simulink library "CRYP_TM_MASTER"  (Simulink 8.6)
settings: Solver=ode45  StartTime=0.0  StopTime=10.0  RelTol=1e-3
libraries: cdsEpicsOut x49, cdsTP x16, VIS_LIB x11, cdsFilt x5, cdsFunctionCall x5, cdsEpicsBinIn x4, cdsFiltCtrl x4, CRYP_TM_MASTER x4, cdsMuxMatrix x3, QPD x2, KAGRA_UTIL x1, cdsEpicsIn x1
(part 1 of 2)
settings Model: Creator=controls  LastModifiedBy=controls

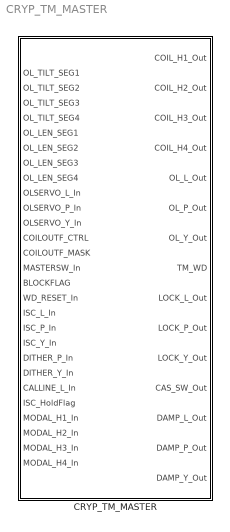
== system CRYP_TM_MASTER ==
  CRYP_TM_MASTER : Subsystem

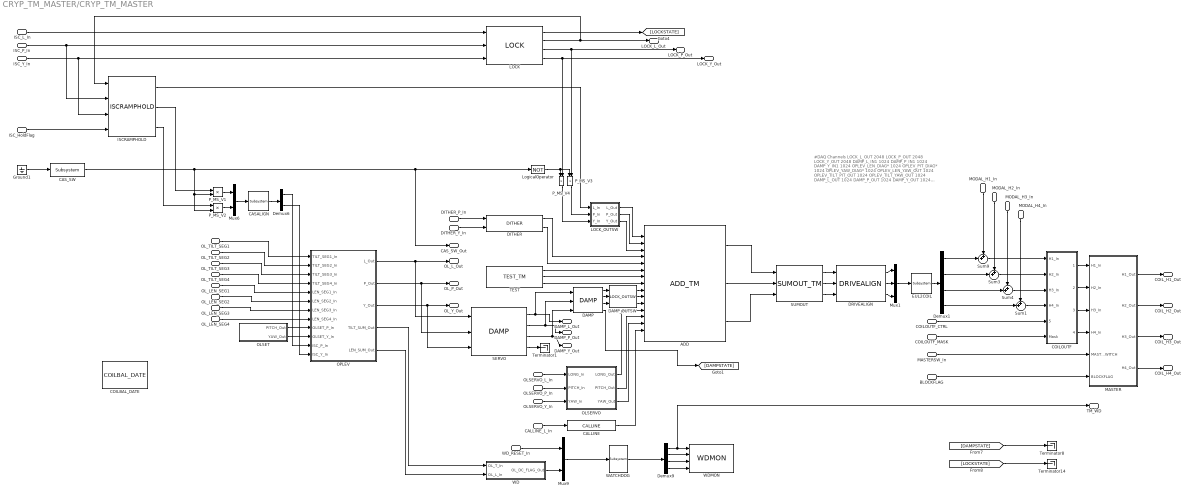
== system CRYP_TM_MASTER/CRYP_TM_MASTER ==
  note: #DAQ Channels
      | LOCK_L_OUT 2048
      | LOCK_P_OUT 2048
      | LOCK_Y_OUT 2048
      | DAMP_L_IN1 1024
      | DAMP_P_IN1 1024
      | DAMP_Y_IN1 1024
      | OPLEV_LEN_DIAG* 1024
      | OPLEV_PIT_DIAG* 1024
      | OPLEV_YAW_DIAG* 1024
      | OPLEV_LEN_YAW_OUT 1024
      | OPLEV_TILT_PIT_OUT 1024
      | OPLEV_TILT_YAW_OUT 1024
      | DAMP_L_OUT 1024
      | DAMP_P_OUT 1024
      | DAMP_Y_OUT 1024
      | MASTER_OUT_H1 1024
      | MASTER_OUT_H2 1024
      | MASTER_OUT_H3 1024
      | MASTER_OUT_H4 1024
      | SUMOUT_L_OUT 512
      | SUMOUT_P_OUT 512
      | SUMOUT_Y_OUT 512
  OL_TILT_SEG1 : Inport
  OL_TILT_SEG2 : Inport  Port=2
  OL_TILT_SEG3 : Inport  Port=3
  OL_TILT_SEG4 : Inport  Port=4
  OL_LEN_SEG1 : Inport  Port=5
  OL_LEN_SEG2 : Inport  Port=6
  OL_LEN_SEG3 : Inport  Port=7
  OL_LEN_SEG4 : Inport  Port=8
  OLSERVO_L_In : Inport  Port=9
  OLSERVO_P_In : Inport  Port=10
  OLSERVO_Y_In : Inport  Port=11
  COILOUTF_CTRL : Inport  Port=12
  COILOUTF_MASK : Inport  Port=13
  MASTERSW_In : Inport  Port=14
  BLOCKFLAG : Inport  Port=15
  WD_RESET_In : Inport  Port=16
  ISC_L_In : Inport  Port=17
  ISC_P_In : Inport  Port=18
  ISC_Y_In : Inport  Port=19
  DITHER_P_In : Inport  Port=20
  DITHER_Y_In : Inport  Port=21
  CALLINE_L_In : Inport  Port=22
  ISC_HoldFlag : Inport  Port=23
  MODAL_H1_In : Inport  Port=24
  MODAL_H2_In : Inport  Port=25
  MODAL_H3_In : Inport  Port=26
  MODAL_H4_In : Inport  Port=27
  ADD : VIS_LIB/CrypParts/ADD_TM
  CALLINE : VIS_LIB/CALLINE
  CASALIGN : cdsMuxMatrix/Subsystem  Tag=cdsMuxMatrix  Description=Any size matrix. Inputs and outputs must be connected using Mux and Demux parts.
      settings: AttributesFormatString=%<Tag>
  CAS_SW : cdsEpicsBinIn/Subsystem  Tag=cdsEpicsBinIn  Description=|
      | Purpose:                                                                            
      | Create an EPICS binary (0 or 1) input channel to the FE realtime controls.          
      |                                                                                     
      | Operation:                                                                          
      | Outputs value from an EPICS ai record. Value is binary input (bi Epics record type).
      |                                                                                     
      | Usage:                                                                              
      | Name the part with the desired EPICS channel name.
      settings: AttributesFormatString=%<Tag>
  COILBAL_DATE : VIS_LIB/COILBAL_DATE
  COILOUTF : Subsystem
  DAMP : VIS_LIB/DAMP
  DAMP_OUTSW : CRYP_TM_MASTER/CRYP_TM_MASTER/LOCK_OUTSW
  DITHER : VIS_LIB/DITHER
  DRIVEALIGN : VIS_LIB/CrypParts/DRIVEALIGN
  Demux1 : Demux
  Demux6 : Demux  Outputs=2
  Demux9 : Demux
  EUL2COIL : cdsMuxMatrix/Subsystem  Tag=cdsMuxMatrix  Description=Any size matrix. Inputs and outputs must be connected using Mux and Demux parts.
      settings: AttributesFormatString=%<Tag>
  Ground1 : Ground
  ISCRAMPHOLD : KAGRA_UTIL/ISCRAMPHOLD
  LOCK : VIS_LIB/LOCK
  LOCK_OUTSW : Subsystem
  LogicalOperator : Logic  Operator=NOT  AllPortsSameDT=off  OutDataTypeStr=boolean
  MASTER : Subsystem
  Mux1 : Mux  Inputs=3
  Mux6 : Mux  Inputs=2
  Mux9 : Mux  Inputs=2
  OLSERVO : Subsystem
  OLSET : Subsystem
  OPLEV : Subsystem
  P_MS_V{1..4} (4 alike) : Product  RndMeth=Zero
  SERVO : VIS_LIB/DAMP
  SUMOUT : VIS_LIB/CrypParts/SUMOUT_TM
  Sum{1,3..4,9} (4 alike) : Sum  Inputs=++|
  TEST : VIS_LIB/CrypParts/TEST_TM
  Terminator1 : Terminator
  Terminator14 : Terminator
  Terminator8 : Terminator
  WATCHDOG : cdsFunctionCall/Subsystem  Tag=cdsFunctionCall  Description=inline OSEMWATCHDOG /opt/rtcds/userapps/release/vis/common/src/WATCHDOG.c
      settings: AttributesFormatString=%<Tag>\n%<Description>
  WD : Subsystem
  WDMON : VIS_LIB/WDMON
  COIL_H1_Out : Outport
  COIL_H2_Out : Outport  Port=2
  COIL_H3_Out : Outport  Port=3
  COIL_H4_Out : Outport  Port=4
  OL_L_Out : Outport  Port=5
  OL_P_Out : Outport  Port=6
  OL_Y_Out : Outport  Port=7
  TM_WD : Outport  Port=8
  LOCK_L_Out : Outport  Port=9
  LOCK_P_Out : Outport  Port=10
  LOCK_Y_Out : Outport  Port=11
  CAS_SW_Out : Outport  Port=12
  DAMP_L_Out : Outport  Port=13
  DAMP_P_Out : Outport  Port=14
  DAMP_Y_Out : Outport  Port=15
  wires:
  ADD/3 -> SUMOUT/3
  ADD/2 -> SUMOUT/2
  ADD/1 -> SUMOUT/1
  Demux1/4 -> Sum1/2
  MODAL_H4_In/1 -> Sum1/1
  Sum1/1 -> COILOUTF/4(H4_In)
  Demux1/3 -> Sum4/2
  Demux1/2 -> Sum3/2
  MODAL_H3_In/1 -> Sum4/1
  Sum4/1 -> COILOUTF/3(H3_In)
  MODAL_H2_In/1 -> Sum3/1
  Sum3/1 -> COILOUTF/2(H2_In)
  Demux1/1 -> Sum9/2
  MODAL_H1_In/1 -> Sum9/1
  Sum9/1 -> COILOUTF/1(H1_In)
  ISC_P_In/1 -> LOCK/2, ISCRAMPHOLD/2
  ISCRAMPHOLD/1 -> LOCK_OUTSW/1(L_In)
  ISCRAMPHOLD/3 -> P_MS_V2/1
  ISCRAMPHOLD/2 -> P_MS_V1/1
  ISC_HoldFlag/1 -> ISCRAMPHOLD/4
  ISC_Y_In/1 -> LOCK/3, ISCRAMPHOLD/3
  LOCK/2 -> ISCRAMPHOLD/1, LOCK_L_Out/1
  OL_TILT_SEG3/1 -> OPLEV/3(TILT_SEG3_In)
  OL_LEN_SEG4/1 -> OPLEV/8(LEN_SEG4_In)
  OL_LEN_SEG3/1 -> OPLEV/7(LEN_SEG3_In)
  OL_LEN_SEG2/1 -> OPLEV/6(LEN_SEG2_In)
  OL_LEN_SEG1/1 -> OPLEV/5(LEN_SEG1_In)
  OL_TILT_SEG4/1 -> OPLEV/4(TILT_SEG4_In)
  OL_TILT_SEG2/1 -> OPLEV/2(TILT_SEG2_In)
  OL_TILT_SEG1/1 -> OPLEV/1(TILT_SEG1_In)
  COILOUTF_CTRL/1 -> COILOUTF/5(Control)
  COILOUTF_MASK/1 -> COILOUTF/6(Mask)
  WD_RESET_In/1 -> Mux9/1
  COILOUTF/4(H4_Out) -> MASTER/4(H4_In)
  COILOUTF/3(H3_Out) -> MASTER/3(H3_In)
  COILOUTF/2(H2_Out) -> MASTER/2(H2_In)
  COILOUTF/1(H1_Out) -> MASTER/1(H1_In)
  Demux9/1 -> TM_WD/1, WDMON/1
  Mux9/1 -> WATCHDOG/1
  WATCHDOG/1 -> Demux9/1
  Demux9/4 -> WDMON/4
  Demux9/3 -> WDMON/3
  Demux9/2 -> WDMON/2
  EUL2COIL/1 -> Demux1/1
  Mux1/1 -> EUL2COIL/1
  DITHER_P_In/1 -> DITHER/1
  DITHER_Y_In/1 -> DITHER/2
  MASTER/1(H1_Out) -> COIL_H1_Out/1
  MASTER/2(H2_Out) -> COIL_H2_Out/1
  MASTER/3(H3_Out) -> COIL_H3_Out/1
  MASTER/4(H4_Out) -> COIL_H4_Out/1
  MASTERSW_In/1 -> MASTER/5(MASTERSWITCH)
  [DAMPSTATE] -> Terminator8/1
  [LOCKSTATE] -> Terminator14/1
  LOCK/1 -> [LOCKSTATE]
  WD/1(OL_DC_FLAG_Out) -> Mux9/2
  ISC_L_In/1 -> LOCK/1
  BLOCKFLAG/1 -> MASTER/6(BLOCKFLAG)
  OPLEV/1(L_Out) -> SERVO/1, OL_L_Out/1
  OPLEV/2(P_Out) -> SERVO/2, OL_P_Out/1
  OPLEV/3(Y_Out) -> SERVO/3, OL_Y_Out/1
  OPLEV/4(TILT_SUM_Out) -> WD/1(OL_T_In)
  OPLEV/5(LEN_SUM_Out) -> WD/2(OL_L_In)
  LOCK/4 -> LOCK_Y_Out/1, P_MS_V4/2
  LOCK/3 -> LOCK_P_Out/1, P_MS_V3/2
  DITHER/2 -> ADD/5
  DITHER/1 -> ADD/4
  TEST/3 -> ADD/8
  TEST/2 -> ADD/7
  TEST/1 -> ADD/6
  SERVO/2 -> DAMP/2, DAMP_P_Out/1
  SERVO/3 -> DAMP/3, DAMP_Y_Out/1
  SUMOUT/2 -> DRIVEALIGN/2
  SUMOUT/1 -> DRIVEALIGN/1
  SUMOUT/3 -> DRIVEALIGN/3
  DRIVEALIGN/3 -> Mux1/3
  DRIVEALIGN/1 -> Mux1/1
  DRIVEALIGN/2 -> Mux1/2
  OLSERVO_L_In/1 -> OLSERVO/1(LONG_In)
  OLSERVO_P_In/1 -> OLSERVO/2(PITCH_In)
  OLSERVO_Y_In/1 -> OLSERVO/3(YAW_In)
  OLSERVO/1(LONG_Out) -> ADD/12
  OLSERVO/2(PITCH_Out) -> ADD/13
  OLSERVO/3(YAW_Out) -> ADD/14
  LOCK_OUTSW/1(L_Out) -> ADD/1
  LOCK_OUTSW/2(P_Out) -> ADD/2
  LOCK_OUTSW/3(Y_Out) -> ADD/3
  OLSET/1(PITCH_Out) -> OPLEV/9(OLSET_P_In)
  OLSET/2(YAW_Out) -> OPLEV/10(OLSET_Y_In)
  Ground1/1 -> CAS_SW/1
  P_MS_V1/1 -> Mux6/1
  P_MS_V2/1 -> Mux6/2
  Mux6/1 -> CASALIGN/1
  CASALIGN/1 -> Demux6/1
  Demux6/1 -> OPLEV/11(ISC_P_In)
  Demux6/2 -> OPLEV/12(ISC_Y_In)
  P_MS_V4/1 -> LOCK_OUTSW/3(Y_In)
  P_MS_V3/1 -> LOCK_OUTSW/2(P_In)
  LogicalOperator/1 -> P_MS_V4/1, P_MS_V3/1
  CAS_SW/1 -> P_MS_V2/2, P_MS_V1/2, CAS_SW_Out/1, LogicalOperator/1
  SERVO/1 -> DAMP/1, DAMP_L_Out/1
  DAMP_OUTSW/1 -> ADD/9
  DAMP_OUTSW/2 -> ADD/10
  DAMP_OUTSW/3 -> ADD/11
  SERVO/4 -> Terminator1/1
  DAMP/4 -> [DAMPSTATE]
  DAMP/1 -> DAMP_OUTSW/1
  DAMP/2 -> DAMP_OUTSW/2
  DAMP/3 -> DAMP_OUTSW/3
  CALLINE_L_In/1 -> CALLINE/1
  CALLINE/1 -> ADD/15

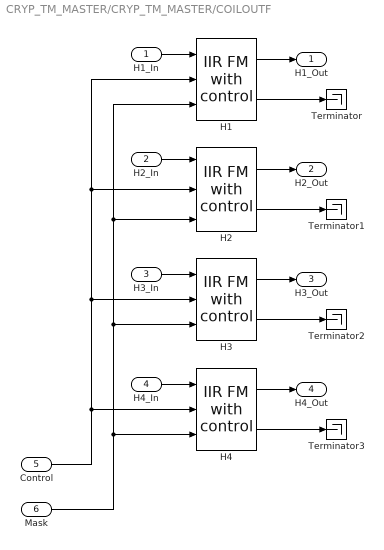
== system CRYP_TM_MASTER/CRYP_TM_MASTER/COILOUTF ==
  H1_In : Inport
  H2_In : Inport  Port=2
  H3_In : Inport  Port=3
  H4_In : Inport  Port=4
  Control : Inport  Port=5
  Mask : Inport  Port=6
  H1 : cdsFiltCtrl/IIR FM with control  Tag=cdsFiltCtrl  Description=|
      | cdsFiltCntrl is the standard IIR filter module (exactly the same as cdsFilt) but with added control data output 'Ctrl'. Filter module digital signal output appears on the first output, which is called 'Val'. 'Ctrl' output has a bit pattern encoding the state of filter's on/off switches (FM1 through FM10). The bit values are:
      |                                                                                                                                                                                                                                                                                                                                       
      | module 	hex	dec                                                                                                                                                                                                                                                                                                                       
      | -----------------------                                                                                                                                                                                                                                                                                                               
      | FM1	0x20                    32                                                                                                                                                                                                                                                                                                        
      | FM2	0x80                     128                                                                                                                                                                                                                                                                                                      
      | FM3	0x200                   512                                                                                                                                                                                                                                                                                                       
      | FM4	0x800                   2048                                                                                                                                                                                                                                                                                                      
      | FM5	0x2000                 8192                                                                                                                                                                                                                                                                                                       
      | FM6	0x8000                 32768                                                                                                                                                                                                                                                                                                      
      | FM7	0x20000                131072                                                                                                                                                                                                                                                                                                     
      | FM8	0x80000                 524288                                                                                                                                                                                                                                                                                                    
      | FM9	0x200000               2097152                                                                                                                                                                                                                                                                                                    
      | FM10	0x800000               8388608                                                                                                                                                                                                                                                                                                   
      |                                                                                                                                                                                                                                                                                                                                       
      | This bit data can be used to drive some other switches or it can be output using a binary I/O module.
      settings: AttributesFormatString=%<Tag>
  H2 : cdsFiltCtrl/IIR FM with control  Tag=cdsFiltCtrl  Description=|
      | cdsFiltCntrl is the standard IIR filter module (exactly the same as cdsFilt) but with added control data output 'Ctrl'. Filter module digital signal output appears on the first output, which is called 'Val'. 'Ctrl' output has a bit pattern encoding the state of filter's on/off switches (FM1 through FM10). The bit values are:
      |                                                                                                                                                                                                                                                                                                                                       
      | module 	hex	dec                                                                                                                                                                                                                                                                                                                       
      | -----------------------                                                                                                                                                                                                                                                                                                               
      | FM1	0x20                    32                                                                                                                                                                                                                                                                                                        
      | FM2	0x80                     128                                                                                                                                                                                                                                                                                                      
      | FM3	0x200                   512                                                                                                                                                                                                                                                                                                       
      | FM4	0x800                   2048                                                                                                                                                                                                                                                                                                      
      | FM5	0x2000                 8192                                                                                                                                                                                                                                                                                                       
      | FM6	0x8000                 32768                                                                                                                                                                                                                                                                                                      
      | FM7	0x20000                131072                                                                                                                                                                                                                                                                                                     
      | FM8	0x80000                 524288                                                                                                                                                                                                                                                                                                    
      | FM9	0x200000               2097152                                                                                                                                                                                                                                                                                                    
      | FM10	0x800000               8388608                                                                                                                                                                                                                                                                                                   
      |                                                                                                                                                                                                                                                                                                                                       
      | This bit data can be used to drive some other switches or it can be output using a binary I/O module.
      settings: AttributesFormatString=%<Tag>
  H3 : cdsFiltCtrl/IIR FM with control  Tag=cdsFiltCtrl  Description=|
      | cdsFiltCntrl is the standard IIR filter module (exactly the same as cdsFilt) but with added control data output 'Ctrl'. Filter module digital signal output appears on the first output, which is called 'Val'. 'Ctrl' output has a bit pattern encoding the state of filter's on/off switches (FM1 through FM10). The bit values are:
      |                                                                                                                                                                                                                                                                                                                                       
      | module 	hex	dec                                                                                                                                                                                                                                                                                                                       
      | -----------------------                                                                                                                                                                                                                                                                                                               
      | FM1	0x20                    32                                                                                                                                                                                                                                                                                                        
      | FM2	0x80                     128                                                                                                                                                                                                                                                                                                      
      | FM3	0x200                   512                                                                                                                                                                                                                                                                                                       
      | FM4	0x800                   2048                                                                                                                                                                                                                                                                                                      
      | FM5	0x2000                 8192                                                                                                                                                                                                                                                                                                       
      | FM6	0x8000                 32768                                                                                                                                                                                                                                                                                                      
      | FM7	0x20000                131072                                                                                                                                                                                                                                                                                                     
      | FM8	0x80000                 524288                                                                                                                                                                                                                                                                                                    
      | FM9	0x200000               2097152                                                                                                                                                                                                                                                                                                    
      | FM10	0x800000               8388608                                                                                                                                                                                                                                                                                                   
      |                                                                                                                                                                                                                                                                                                                                       
      | This bit data can be used to drive some other switches or it can be output using a binary I/O module.
      settings: AttributesFormatString=%<Tag>
  H4 : cdsFiltCtrl/IIR FM with control  Tag=cdsFiltCtrl  Description=|
      | cdsFiltCntrl is the standard IIR filter module (exactly the same as cdsFilt) but with added control data output 'Ctrl'. Filter module digital signal output appears on the first output, which is called 'Val'. 'Ctrl' output has a bit pattern encoding the state of filter's on/off switches (FM1 through FM10). The bit values are:
      |                                                                                                                                                                                                                                                                                                                                       
      | module 	hex	dec                                                                                                                                                                                                                                                                                                                       
      | -----------------------                                                                                                                                                                                                                                                                                                               
      | FM1	0x20                    32                                                                                                                                                                                                                                                                                                        
      | FM2	0x80                     128                                                                                                                                                                                                                                                                                                      
      | FM3	0x200                   512                                                                                                                                                                                                                                                                                                       
      | FM4	0x800                   2048                                                                                                                                                                                                                                                                                                      
      | FM5	0x2000                 8192                                                                                                                                                                                                                                                                                                       
      | FM6	0x8000                 32768                                                                                                                                                                                                                                                                                                      
      | FM7	0x20000                131072                                                                                                                                                                                                                                                                                                     
      | FM8	0x80000                 524288                                                                                                                                                                                                                                                                                                    
      | FM9	0x200000               2097152                                                                                                                                                                                                                                                                                                    
      | FM10	0x800000               8388608                                                                                                                                                                                                                                                                                                   
      |                                                                                                                                                                                                                                                                                                                                       
      | This bit data can be used to drive some other switches or it can be output using a binary I/O module.
      settings: AttributesFormatString=%<Tag>
  Terminator{,1..3} (4 alike) : Terminator
  H1_Out : Outport
  H2_Out : Outport  Port=2
  H3_Out : Outport  Port=3
  H4_Out : Outport  Port=4
  wires:
  H1/1 -> H1_Out/1
  H1_In/1 -> H1/1
  H2_In/1 -> H2/1
  H2/1 -> H2_Out/1
  H3_In/1 -> H3/1
  H3/1 -> H3_Out/1
  H4_In/1 -> H4/1
  H4/1 -> H4_Out/1
  H1/2 -> Terminator/1
  H2/2 -> Terminator1/1
  H4/2 -> Terminator3/1
  H3/2 -> Terminator2/1
  Mask/1 -> H4/3, H3/3, H2/3, H1/3
  Control/1 -> H4/2, H3/2, H2/2, H1/2

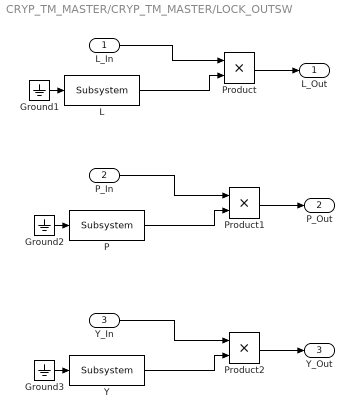
== system CRYP_TM_MASTER/CRYP_TM_MASTER/LOCK_OUTSW ==
  L_In : Inport
  P_In : Inport  Port=2
  Y_In : Inport  Port=3
  Ground1 : Ground
  Ground2 : Ground
  Ground3 : Ground
  L : cdsEpicsBinIn/Subsystem  Tag=cdsEpicsBinIn  Description=|
      | Purpose:                                                                            
      | Create an EPICS binary (0 or 1) input channel to the FE realtime controls.          
      |                                                                                     
      | Operation:                                                                          
      | Outputs value from an EPICS ai record. Value is binary input (bi Epics record type).
      |                                                                                     
      | Usage:                                                                              
      | Name the part with the desired EPICS channel name.
      settings: AttributesFormatString=%<Tag>
  P : cdsEpicsBinIn/Subsystem  Tag=cdsEpicsBinIn  Description=|
      | Purpose:                                                                            
      | Create an EPICS binary (0 or 1) input channel to the FE realtime controls.          
      |                                                                                     
      | Operation:                                                                          
      | Outputs value from an EPICS ai record. Value is binary input (bi Epics record type).
      |                                                                                     
      | Usage:                                                                              
      | Name the part with the desired EPICS channel name.
      settings: AttributesFormatString=%<Tag>
  Product : Product  RndMeth=Zero
  Product1 : Product  RndMeth=Zero
  Product2 : Product  RndMeth=Zero
  Y : cdsEpicsBinIn/Subsystem  Tag=cdsEpicsBinIn  Description=|
      | Purpose:                                                                            
      | Create an EPICS binary (0 or 1) input channel to the FE realtime controls.          
      |                                                                                     
      | Operation:                                                                          
      | Outputs value from an EPICS ai record. Value is binary input (bi Epics record type).
      |                                                                                     
      | Usage:                                                                              
      | Name the part with the desired EPICS channel name.
      settings: AttributesFormatString=%<Tag>
  L_Out : Outport
  P_Out : Outport  Port=2
  Y_Out : Outport  Port=3
  wires:
  L_In/1 -> Product/1
  Product/1 -> L_Out/1
  Ground1/1 -> L/1
  L/1 -> Product/2
  Ground2/1 -> P/1
  P/1 -> Product1/2
  P_In/1 -> Product1/1
  Product1/1 -> P_Out/1
  Ground3/1 -> Y/1
  Y/1 -> Product2/2
  Y_In/1 -> Product2/1
  Product2/1 -> Y_Out/1

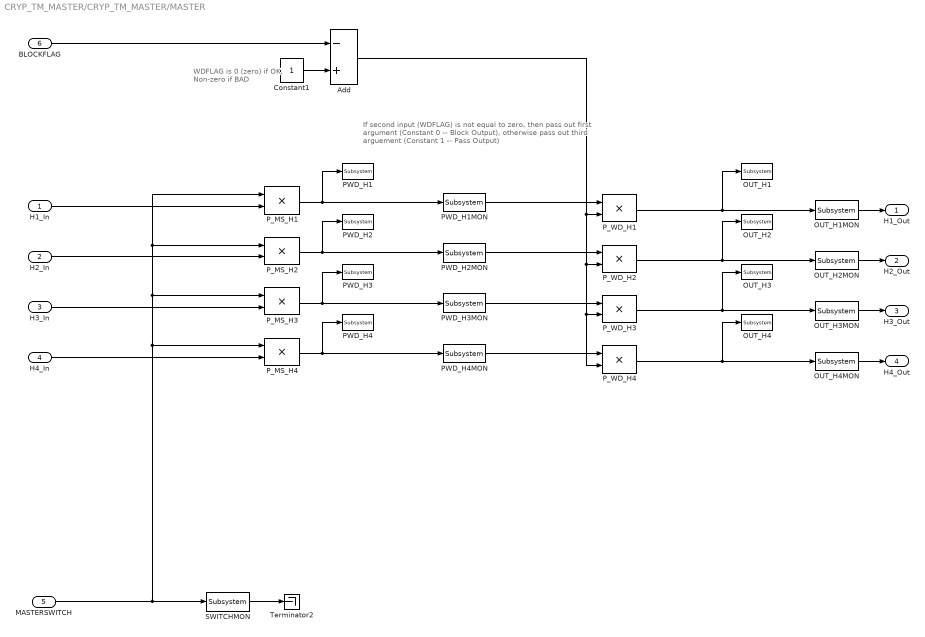
== system CRYP_TM_MASTER/CRYP_TM_MASTER/MASTER ==
  note: WDFLAG is 0 (zero) if OK,
      | Non-zero if BAD
  note: If second input (WDFLAG) is not equal to zero,
      | then pass out first argument (Constant 0 -- Block Output),
      | otherwise pass out third arguement (Constant 1 -- Pass Output)
  H1_In : Inport
  H2_In : Inport  Port=2
  H3_In : Inport  Port=3
  H4_In : Inport  Port=4
  MASTERSWITCH : Inport  Port=5
  BLOCKFLAG : Inport  Port=6
  Add : Sum  Inputs=-+
  Constant1 : Constant
  OUT_H{1..4} (4 alike) : cdsTP/Subsystem  Tag=Test Point
      settings: AttributesFormatString=%<Tag>
  OUT_H1MON : cdsEpicsOut/Subsystem  Tag=cdsEpicsOutput  Description=|
      | Purpose:                                          
      | Output a FE signal to an EPICS channel.           
      |                                                   
      | Operation:                                        
      | Takes input value and passes it to EPICS record.  
      |                                                   
      | Usage:                                            
      | Name the part with the desired EPICS rrecord name.
      settings: AttributesFormatString=%<Tag>
  OUT_H2MON : cdsEpicsOut/Subsystem  Tag=cdsEpicsOutput  Description=|
      | Purpose:                                          
      | Output a FE signal to an EPICS channel.           
      |                                                   
      | Operation:                                        
      | Takes input value and passes it to EPICS record.  
      |                                                   
      | Usage:                                            
      | Name the part with the desired EPICS rrecord name.
      settings: AttributesFormatString=%<Tag>
  OUT_H3MON : cdsEpicsOut/Subsystem  Tag=cdsEpicsOutput  Description=|
      | Purpose:                                          
      | Output a FE signal to an EPICS channel.           
      |                                                   
      | Operation:                                        
      | Takes input value and passes it to EPICS record.  
      |                                                   
      | Usage:                                            
      | Name the part with the desired EPICS rrecord name.
      settings: AttributesFormatString=%<Tag>
  OUT_H4MON : cdsEpicsOut/Subsystem  Tag=cdsEpicsOutput  Description=|
      | Purpose:                                          
      | Output a FE signal to an EPICS channel.           
      |                                                   
      | Operation:                                        
      | Takes input value and passes it to EPICS record.  
      |                                                   
      | Usage:                                            
      | Name the part with the desired EPICS rrecord name.
      settings: AttributesFormatString=%<Tag>
  PWD_H{1..4} (4 alike) : cdsTP/Subsystem  Tag=Test Point
      settings: AttributesFormatString=%<Tag>
  PWD_H1MON : cdsEpicsOut/Subsystem  Tag=cdsEpicsOutput  Description=|
      | Purpose:                                          
      | Output a FE signal to an EPICS channel.           
      |                                                   
      | Operation:                                        
      | Takes input value and passes it to EPICS record.  
      |                                                   
      | Usage:                                            
      | Name the part with the desired EPICS rrecord name.
      settings: AttributesFormatString=%<Tag>
  PWD_H2MON : cdsEpicsOut/Subsystem  Tag=cdsEpicsOutput  Description=|
      | Purpose:                                          
      | Output a FE signal to an EPICS channel.           
      |                                                   
      | Operation:                                        
      | Takes input value and passes it to EPICS record.  
      |                                                   
      | Usage:                                            
      | Name the part with the desired EPICS rrecord name.
      settings: AttributesFormatString=%<Tag>
  PWD_H3MON : cdsEpicsOut/Subsystem  Tag=cdsEpicsOutput  Description=|
      | Purpose:                                          
      | Output a FE signal to an EPICS channel.           
      |                                                   
      | Operation:                                        
      | Takes input value and passes it to EPICS record.  
      |                                                   
      | Usage:                                            
      | Name the part with the desired EPICS rrecord name.
      settings: AttributesFormatString=%<Tag>
  PWD_H4MON : cdsEpicsOut/Subsystem  Tag=cdsEpicsOutput  Description=|
      | Purpose:                                          
      | Output a FE signal to an EPICS channel.           
      |                                                   
      | Operation:                                        
      | Takes input value and passes it to EPICS record.  
      |                                                   
      | Usage:                                            
      | Name the part with the desired EPICS rrecord name.
      settings: AttributesFormatString=%<Tag>
  P_MS_H{1..4} (4 alike) : Product  RndMeth=Zero
  P_WD_H{1..4} (4 alike) : Product  RndMeth=Zero
  SWITCHMON : cdsEpicsOut/Subsystem  Tag=cdsEpicsOutput  Description=|
      | Purpose:                                          
      | Output a FE signal to an EPICS channel.           
      |                                                   
      | Operation:                                        
      | Takes input value and passes it to EPICS record.  
      |                                                   
      | Usage:                                            
      | Name the part with the desired EPICS rrecord name.
      settings: AttributesFormatString=%<Tag>
  Terminator2 : Terminator
  H1_Out : Outport
  H2_Out : Outport  Port=2
  H3_Out : Outport  Port=3
  H4_Out : Outport  Port=4
  wires:
  SWITCHMON/1 -> Terminator2/1
  BLOCKFLAG/1 -> Add/1
  Constant1/1 -> Add/2
  P_WD_H4/1 -> OUT_H4/1, OUT_H4MON/1
  P_WD_H3/1 -> OUT_H3/1, OUT_H3MON/1
  P_WD_H2/1 -> OUT_H2/1, OUT_H2MON/1
  P_WD_H1/1 -> OUT_H1/1, OUT_H1MON/1
  P_MS_H4/1 -> PWD_H4/1, PWD_H4MON/1
  P_MS_H3/1 -> PWD_H3/1, PWD_H3MON/1
  P_MS_H2/1 -> PWD_H2/1, PWD_H2MON/1
  P_MS_H1/1 -> PWD_H1/1, PWD_H1MON/1
  OUT_H4MON/1 -> H4_Out/1
  OUT_H3MON/1 -> H3_Out/1
  OUT_H1MON/1 -> H1_Out/1
  OUT_H2MON/1 -> H2_Out/1
  MASTERSWITCH/1 -> SWITCHMON/1, P_MS_H1/1, P_MS_H2/1, P_MS_H3/1, P_MS_H4/1
  H4_In/1 -> P_MS_H4/2
  H3_In/1 -> P_MS_H3/2
  H2_In/1 -> P_MS_H2/2
  H1_In/1 -> P_MS_H1/2
  PWD_H1MON/1 -> P_WD_H1/1
  PWD_H2MON/1 -> P_WD_H2/1
  PWD_H3MON/1 -> P_WD_H3/1
  PWD_H4MON/1 -> P_WD_H4/1
  Add/1 -> P_WD_H4/2, P_WD_H3/2, P_WD_H2/2, P_WD_H1/2

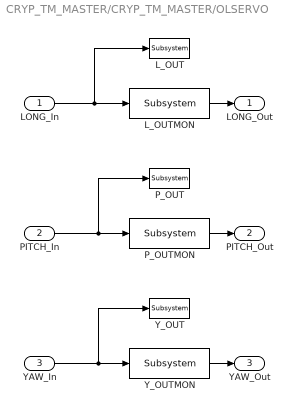
== system CRYP_TM_MASTER/CRYP_TM_MASTER/OLSERVO ==
  LONG_In : Inport
  PITCH_In : Inport  Port=2
  YAW_In : Inport  Port=3
  L_OUT : cdsTP/Subsystem  Tag=Test Point
      settings: AttributesFormatString=%<Tag>
  L_OUTMON : cdsEpicsOut/Subsystem  Tag=cdsEpicsOutput  Description=|
      | Purpose:                                          
      | Output a FE signal to an EPICS channel.           
      |                                                   
      | Operation:                                        
      | Takes input value and passes it to EPICS record.  
      |                                                   
      | Usage:                                            
      | Name the part with the desired EPICS rrecord name.
      settings: AttributesFormatString=%<Tag>
  P_OUT : cdsTP/Subsystem  Tag=Test Point
      settings: AttributesFormatString=%<Tag>
  P_OUTMON : cdsEpicsOut/Subsystem  Tag=cdsEpicsOutput  Description=|
      | Purpose:                                          
      | Output a FE signal to an EPICS channel.           
      |                                                   
      | Operation:                                        
      | Takes input value and passes it to EPICS record.  
      |                                                   
      | Usage:                                            
      | Name the part with the desired EPICS rrecord name.
      settings: AttributesFormatString=%<Tag>
  Y_OUT : cdsTP/Subsystem  Tag=Test Point
      settings: AttributesFormatString=%<Tag>
  Y_OUTMON : cdsEpicsOut/Subsystem  Tag=cdsEpicsOutput  Description=|
      | Purpose:                                          
      | Output a FE signal to an EPICS channel.           
      |                                                   
      | Operation:                                        
      | Takes input value and passes it to EPICS record.  
      |                                                   
      | Usage:                                            
      | Name the part with the desired EPICS rrecord name.
      settings: AttributesFormatString=%<Tag>
  LONG_Out : Outport
  PITCH_Out : Outport  Port=2
  YAW_Out : Outport  Port=3
  wires:
  L_OUTMON/1 -> LONG_Out/1
  LONG_In/1 -> L_OUT/1, L_OUTMON/1
  P_OUTMON/1 -> PITCH_Out/1
  PITCH_In/1 -> P_OUT/1, P_OUTMON/1
  Y_OUTMON/1 -> YAW_Out/1
  YAW_In/1 -> Y_OUT/1, Y_OUTMON/1

== system CRYP_TM_MASTER/CRYP_TM_MASTER/OLSET ==
  Ground1 : Ground
  Ground2 : Ground
  P : cdsFilt/Subsystem  Tag=cdsFilt  Description=|
      | Purpose:                                                                                                                                                                                                                                  
      | Standard CDS IIR filter module.                                                                                                                                                                                                           
      |                                                                                                                                                                                                                                           
      | Operation:                                                                                                                                                                                                                                
      | Consists of 10 second order section IIR filters, plus a ramped gain stage. In FE code, also provides pre-defined test points and excitation channel inputs. The filter coefficients are defined in the LIGO system using the 'foton' tool.
      |                                                                                                                                                                                                                                           
      | Usage:                                                                                                                                                                                                                                    
      | Name the part with the desired filter module name.
      settings: AttributesFormatString=%<Tag>
  Y : cdsFilt/Subsystem  Tag=cdsFilt  Description=|
      | Purpose:                                                                                                                                                                                                                                  
      | Standard CDS IIR filter module.                                                                                                                                                                                                           
      |                                                                                                                                                                                                                                           
      | Operation:                                                                                                                                                                                                                                
      | Consists of 10 second order section IIR filters, plus a ramped gain stage. In FE code, also provides pre-defined test points and excitation channel inputs. The filter coefficients are defined in the LIGO system using the 'foton' tool.
      |                                                                                                                                                                                                                                           
      | Usage:                                                                                                                                                                                                                                    
      | Name the part with the desired filter module name.
      settings: AttributesFormatString=%<Tag>
  PITCH_Out : Outport
  YAW_Out : Outport  Port=2
  wires:
  P/1 -> PITCH_Out/1
  Y/1 -> YAW_Out/1
  Ground1/1 -> P/1
  Ground2/1 -> Y/1
